simulink model "EstimateIMUPos"  (R2024b)
settings: Solver=VariableStepAuto  StartTime=0.0  StopTime=inf  RelTol=1e-3
undefined symbols (not defined in the file or in its folder): DiscIntNeverNeededParam
libraries: aerolibanimutils x1, robotcorelib x1
settings Model: Creator=vince  LastModifiedBy=vince

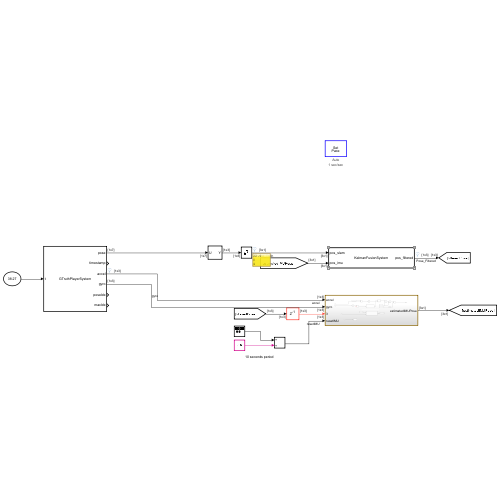
[thumbnail: Simulink's stored preview of the top-level diagram]
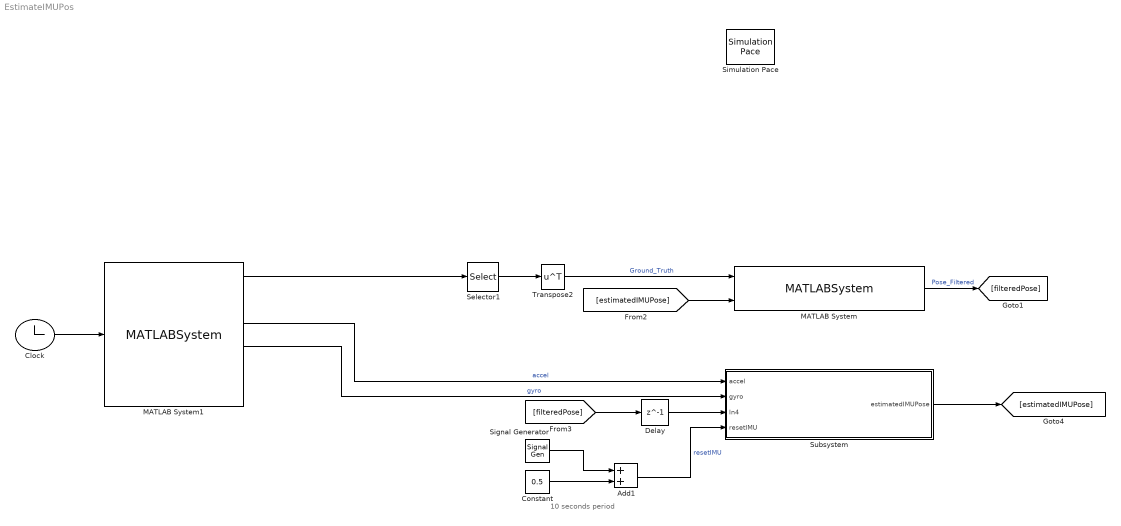
== system EstimateIMUPos ==
  note: 10 seconds period
  Add1 : Sum
  Clock : Clock
  Constant : Constant  Value=0.5
  Delay : Delay  DelayLength=1  InitialCondition=[0 0 0]
  MATLAB System : MATLABSystem  System=KalmanFusionSystem  dt=0.1  noise_std=0.5  Q=0.01 * eye( 6 )  R=diag( [ 0.3, 0.3, 0.3, 1, 1, 1 ] )  SimulateUsing=Interpreted execution
      mask Type: KalmanFusionSystem
      mask Display:
      | disp('KalmanFusionSystem');
      | port_label('input',1,'pos_slam');
      | port_label('input',2,'pos_imu');
      | port_label('output',1,'pos_filtered');
  MATLAB System1 : MATLABSystem  System=GTruthPlayerSystem  groundTruthFile=C:\Users\vince\Documents\SEN5\CollaborativeSLAM\Scenarios\8\uavData.mat  SimulateUsing=Interpreted execution
      mask Type: GTruthPlayerSystem
      mask Display:
      | disp('GTruthPlayerSystem');
      | port_label('input',1,'t');
      | port_label('output',1,'pose');
      | port_label('output',2,'timestamp');
      | port_label('output',3,'accel');
      | port_label('output',4,'gyro');
      | port_label('output',5,'poseIdx');
      | port_label('output',6,'maxIdx');
  Selector1 : Selector  InputPortWidth=7  IndexOptions=Index vector (dialog)  Indices=[1 2 3]  OutputSizes=1
  Signal Generator : SignalGenerator  WaveForm=square  Amplitude=0.5  Frequency=10
  Simulation Pace : aerolibanimutils/Simulation Pace  SimulationPace=1  SleepMode=Auto  OutputPaceError=off  SampleTime=1/30
  Subsystem : Subsystem
  Transpose2 : Math  Operator=transpose
  wires:
  Clock/1 -> MATLAB System1/1
  MATLAB System1/1 -> Selector1/1
  Selector1/1 -> Transpose2/1
  Transpose2/1 -> MATLAB System/1  "Ground_Truth"
  MATLAB System/1 -> [filteredPose]  "Pose_Filtered"
  Signal Generator/1 -> Add1/1
  Constant/1 -> Add1/2
  [estimatedIMUPose] -> MATLAB System/2
  MATLAB System1/3 -> Subsystem/1(accel)  "accel"
  MATLAB System1/4 -> Subsystem/2(gyro)  "gyro"
  [filteredPose] -> Delay/1
  Add1/1 -> Subsystem/4(resetIMU)  "resetIMU"
  Subsystem/1(estimatedIMUPose) -> [estimatedIMUPose]
  Delay/1 -> Subsystem/3(In4)

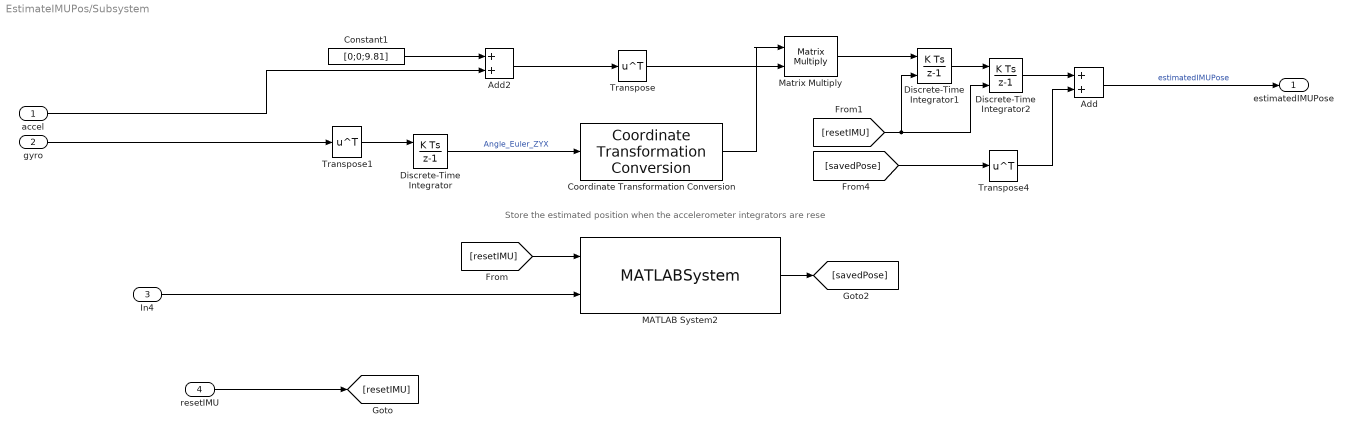
== system EstimateIMUPos/Subsystem ==
  note: Store the estimated position when the accelerometer integrators are rese
  accel : Inport
  gyro : Inport  Port=2
  In4 : Inport  Port=3
  resetIMU : Inport  Port=4
  Add : Sum
  Add2 : Sum
  Constant1 : Constant  Value=[0;0;9.81]
  Coordinate Transformation Conversion : robotcorelib/Coordinate Transformation Conversion  InputRepresentation=Euler Angles  InputEulerSequence=ZYX  ShowTrVecInputPort=on  OutputRepresentation=Rotation Matrix  OutputEulerSequence=ZYX  ShowTrVecOutputPort=on  SimulateUsing=Code generation
      settings: LibrarySourceBlock=navlib/Utilities/Coordinate Transformation Conversion
  Discrete-Time Integrator : DiscreteIntegrator  ExternalReset=rising  SampleTime=0.01  ICPrevOutput=DiscIntNeverNeededParam  ICPrevScaledInput=DiscIntNeverNeededParam
  Discrete-Time Integrator1 : DiscreteIntegrator  ExternalReset=rising  SampleTime=1e-3  ICPrevOutput=DiscIntNeverNeededParam  ICPrevScaledInput=DiscIntNeverNeededParam
  Discrete-Time Integrator2 : DiscreteIntegrator  ExternalReset=rising  SampleTime=1e-3  ICPrevOutput=DiscIntNeverNeededParam  ICPrevScaledInput=DiscIntNeverNeededParam
  MATLAB System2 : MATLABSystem  System=IMUPoseMemory  SimulateUsing=Interpreted execution
      mask Type: IMUPoseMemory
      mask Display:
      | disp('IMUPoseMemory');
      | port_label('input',1,'resetImu');
      | port_label('input',2,'filteredPose');
      | port_label('output',1,'savedPose');
  Matrix Multiply : Product  Multiplication=Matrix(*)
  Transpose : Math  Operator=transpose
  Transpose1 : Math  Operator=transpose
  Transpose4 : Math  Operator=transpose
  estimatedIMUPose : Outport
  wires:
  In4/1 -> MATLAB System2/2
  Transpose1/1 -> Discrete-Time Integrator/1
  [savedPose] -> Transpose4/1
  Constant1/1 -> Add2/1
  Discrete-Time Integrator1/1 -> Discrete-Time Integrator2/1
  ? -> Discrete-Time Integrator/2
  [resetIMU] -> Discrete-Time Integrator1/2, Discrete-Time Integrator2/2
  Matrix Multiply/1 -> Discrete-Time Integrator1/1
  Discrete-Time Integrator2/1 -> Add/1
  Coordinate Transformation Conversion/1 -> Matrix Multiply/1
  Transpose/1 -> Matrix Multiply/2
  Add/1 -> estimatedIMUPose/1  "estimatedIMUPose"
  Discrete-Time Integrator/1 -> Coordinate Transformation Conversion/1  "Angle_Euler_ZYX"
  Add2/1 -> Transpose/1
  Transpose4/1 -> Add/2
  [resetIMU] -> MATLAB System2/1
  MATLAB System2/1 -> [savedPose]
  accel/1 -> Add2/2
  resetIMU/1 -> [resetIMU]
  gyro/1 -> Transpose1/1
